simulink model "InPark"  (R2025b)
settings: Solver=VariableStepAuto  StartTime=0.0  StopTime=10.0  RelTol=1e-3
settings Model: Creator=jff_1  LastModifiedBy=jff_1

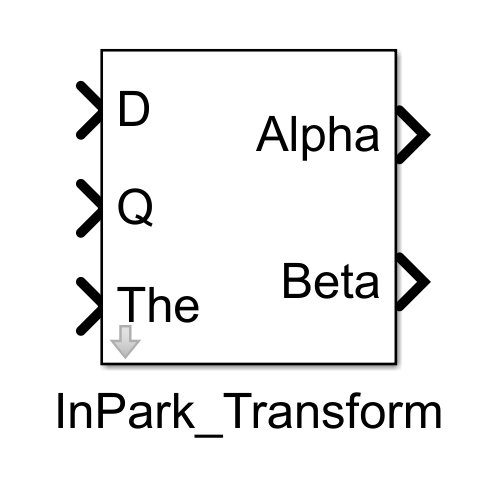
[thumbnail: Simulink's stored preview of the top-level diagram]
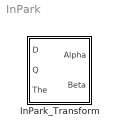
== system InPark ==
  InPark_Transform : Subsystem
      mask help:
      | 反 Park 变换用于将同步旋转坐标系 d–q 中的变量变换回静止坐标系 α–β。
      | 该变换是 Park 变换的逆过程，广泛应用于 PMSM 矢量控制（FOC）中，
      | 用于将 dq 坐标系下的电流或电压还原为 αβ 坐标系量，以便后续调制或坐标变换。
      mask Help:
      | 反 Park 变换的数学表达式为：
      | 
      | [ alpha ]   [ cos(θe)  -sin(θe) ] [ d ]
      | [ beta  ] = [ sin(θe)   cos(θe) ] [ q ]
      | 
      | 即：
      | alpha = d*cos(θe) - q*sin(θe)
      | beta  = d*sin(θe) + q*cos(θe)
      | 
      | 输入端口：
      | D   —— d 轴分量
      | Q   —— q 轴分量
      | The —— 同步旋转角 θe（rad）
      | 
      | 输出端口：
      | Alpha —— α 轴分量
      | Beta  —— β 轴分量
      | 
      | 本模块通常与 Park 变换模块配合使用，
      | 用于 PMSM 矢量控制中 dq → αβ 的坐标变换。
      mask DialogControl ParameterGroupVar Prompt: 参数
      mask Display:
      | % 输入端口标签
      | port_label('input',1,'D');
      | port_label('input',2,'Q');
      | port_label('input',3,'The');
      | 
      | % 输出端口标签
      | port_label('output',1,'Alpha');
      | port_label('output',2,'Beta');

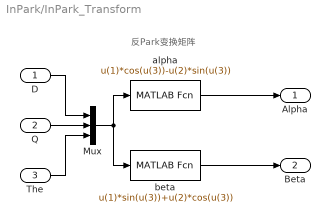
== system InPark/InPark_Transform ==
  note: 反Park变换矩阵
  D : Inport
  Q : Inport  Port=2
  The : Inport  Port=3
  Mux : Mux  Inputs=3
  alpha : MATLABFcn  MATLABFcn=u(1)*cos(u(3))-u(2)*sin(u(3))
  beta : MATLABFcn  MATLABFcn=u(1)*sin(u(3))+u(2)*cos(u(3))
  Alpha : Outport
  Beta : Outport  Port=2
  wires:
  beta/1 -> Beta/1
  The/1 -> Mux/3
  Q/1 -> Mux/2
  Mux/1 -> beta/1, alpha/1
  D/1 -> Mux/1
  alpha/1 -> Alpha/1
